simulink model "Version4"  (R2021a)
settings: Solver=VariableStepAuto  StartTime=0.0  StopTime=10.0  RelTol=1e-3
undefined symbols (not defined in the file): K, Lm, Lr, Rr, Rs
settings Model: Creator=shahk  LastModifiedBy=Aashish Kalra
settings OptimizationCC: UseDivisionForNetSlopeComputation=UseDivisionForReciprocalsOfIntegersOnly  DefaultUnderspecifiedDataType=single
settings DebuggingCC: SignalInfNanChecking=warning  UnconnectedInputMsg=none  UnconnectedOutputMsg=none  UnconnectedLineMsg=none  UniqueDataStoreMsg=error  AssertControl=DisableAll  StrictBusMsg=ErrorOnBusTreatedAsVector
settings SFSimCC: CompileTimeRecursionLimit=0  MATLABDynamicMemAlloc=off
settings RTWCC: DLArmComputeVersion=20.02.1
settings ConfigComp: CovEnable=on  CovScope=ReferencedModels  RecordCoverage=on  CovModelRefEnable=filtered

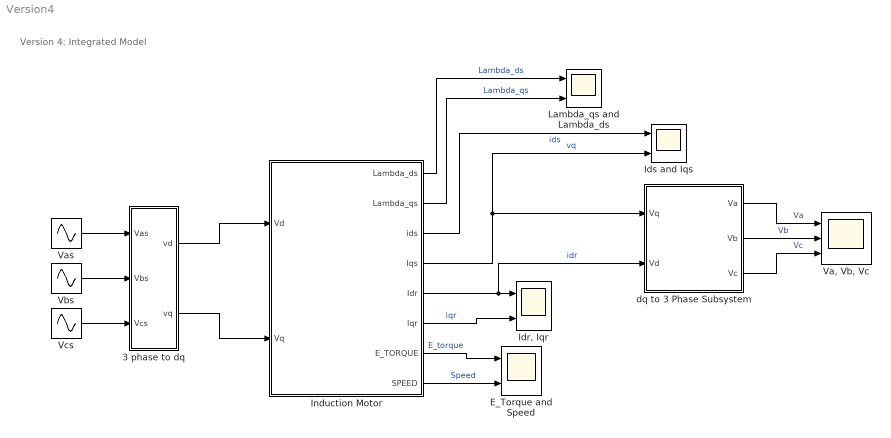
== system Version4 ==
  note: Version 4: Integrated Model
  3 phase to dq : Subsystem
  E_Torque and Speed : Scope  NumInputPorts=2
  "Idr, Iqr" : Scope  NumInputPorts=2
  Ids and Iqs : Scope  NumInputPorts=2
  Induction Motor : Subsystem
  Lambda_qs and Lambda_ds : Scope  NumInputPorts=2
  "Va, Vb, Vc" : Scope  NumInputPorts=3
  Vas : Sin  Amplitude=220*sqrt(2)  Frequency=2*pi*60  Phase=(pi/2)  SampleTime=0
  Vbs : Sin  Amplitude=220*sqrt(2)  Frequency=2*pi*60  Phase=((-2*pi)/3)+(pi/2)  SampleTime=0
  Vcs : Sin  Amplitude=220*sqrt(2)  Frequency=2*pi*60  Phase=((2*pi)/3)+(pi/2)  SampleTime=0
  dq to 3 Phase Subsystem : Subsystem
  wires:
  Induction Motor/6(Iqr) -> "Idr, Iqr"/2  "iqr"
  dq to 3 Phase Subsystem/1(Va) -> "Va, Vb, Vc"/1  "Va"
  dq to 3 Phase Subsystem/3(Vc) -> "Va, Vb, Vc"/3  "Vc"
  Induction Motor/4(Iqs) -> Ids and Iqs/2, dq to 3 Phase Subsystem/1(Vq)  "vq"
  Induction Motor/2(Lambda_qs) -> Lambda_qs and Lambda_ds/2  "Lambda_qs"
  dq to 3 Phase Subsystem/2(Vb) -> "Va, Vb, Vc"/2  "Vb"
  Induction Motor/3(ids) -> Ids and Iqs/1  "ids"
  Induction Motor/8(SPEED) -> E_Torque and Speed/2  "Speed"
  3 phase to dq/2(vq) -> Induction Motor/2(Vq)
  3 phase to dq/1(vd) -> Induction Motor/1(Vd)
  Induction Motor/7("E_TORQUE ") -> E_Torque and Speed/1  "E_torque"
  Induction Motor/5(Idr) -> dq to 3 Phase Subsystem/2(Vd), "Idr, Iqr"/1  "idr"
  Induction Motor/1(Lambda_ds) -> Lambda_qs and Lambda_ds/1  "Lambda_ds"
  Vas/1 -> 3 phase to dq/1(Vas)
  Vbs/1 -> 3 phase to dq/2(Vbs)
  Vcs/1 -> 3 phase to dq/3(Vcs)

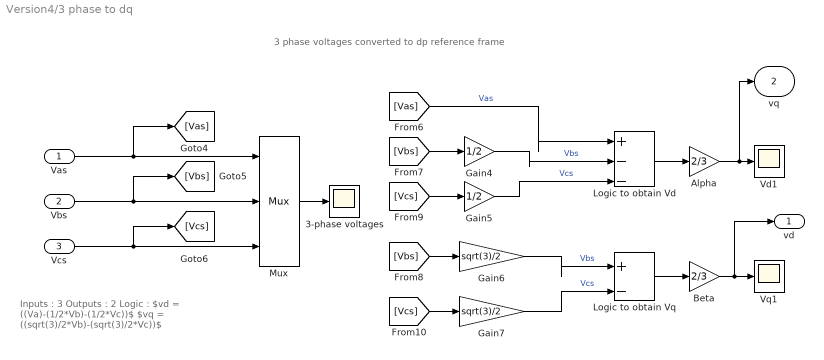
== system Version4/3 phase to dq ==
  note: Inputs : 3
      | Outputs : 2
      |
      | Logic :
      | $vd = ((Va)-(1/2*Vb)-(1/2*Vc))$
      | $vq = ((sqrt(3)/2*Vb)-(sqrt(3)/2*Vc))$
  note: 3 phase voltages converted to dp reference frame
  Vas : Inport
  Vbs : Inport  Port=2
  Vcs : Inport  Port=3
  3-phase voltages : Scope
  Alpha : Gain  Gain=2/3
  Beta : Gain  Gain=2/3
  Gain4 : Gain  Gain=1/2
  Gain5 : Gain  Gain=1/2
  Gain6 : Gain  Gain=sqrt(3)/2
  Gain7 : Gain  Gain=sqrt(3)/2
  Logic to obtain Vd : Sum  Inputs=|+--
  Logic to obtain Vq : Sum  Inputs=|+-
  Mux : Mux  Inputs=3
  Vd1 : Scope
  Vq1 : Scope
  vd : Outport
  vq : Outport  Port=2
  wires:
  Gain4/1 -> Logic to obtain Vd/2  "Vbs"
  Gain7/1 -> Logic to obtain Vq/2  "Vcs"
  [Vcs] -> Gain5/1
  Vcs/1 -> [Vcs], Mux/3
  Vbs/1 -> [Vbs], Mux/2
  [Vas] -> Logic to obtain Vd/1  "Vas"
  Vas/1 -> [Vas], Mux/1
  Logic to obtain Vq/1 -> Beta/1
  [Vcs] -> Gain7/1
  Gain6/1 -> Logic to obtain Vq/1  "Vbs"
  [Vbs] -> Gain6/1
  [Vbs] -> Gain4/1
  Logic to obtain Vd/1 -> Alpha/1
  Gain5/1 -> Logic to obtain Vd/3  "Vcs"
  Beta/1 -> vd/1, Vq1/1
  Mux/1 -> 3-phase voltages/1
  Alpha/1 -> vq/1, Vd1/1

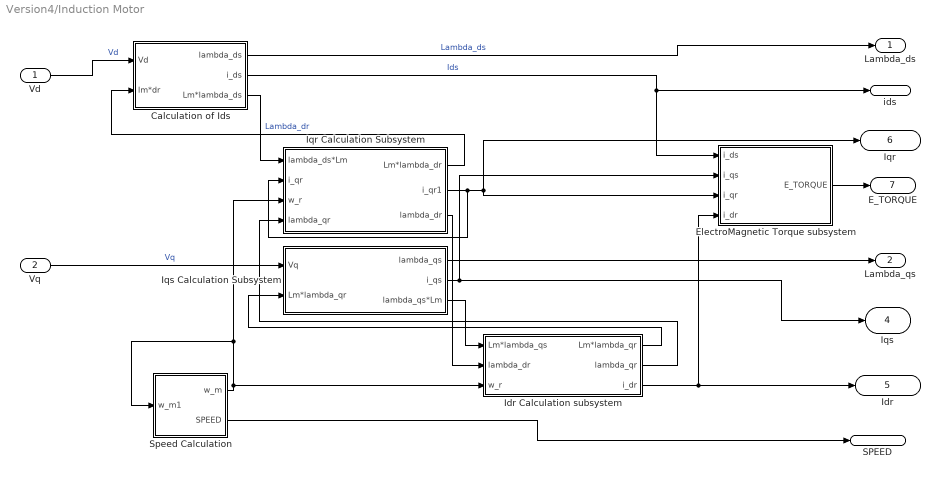
== system Version4/Induction Motor ==
  Vd : Inport
  Vq : Inport  Port=2
  Calculation of Ids : Subsystem
  ElectroMagnetic Torque subsystem : Subsystem
  Idr Calculation subsystem : Subsystem
  Iqr Calculation Subsystem : Subsystem
  Iqs Calculation Subsystem : Subsystem
  Speed Calculation : Subsystem
  Lambda_ds : Outport  VectorParamsAs1DForOutWhenUnconnected=off
  Lambda_qs : Outport  Port=2  VectorParamsAs1DForOutWhenUnconnected=off
  ids : Outport  Port=3  VectorParamsAs1DForOutWhenUnconnected=off
  Iqs : Outport  Port=4  VectorParamsAs1DForOutWhenUnconnected=off
  Idr : Outport  Port=5  VectorParamsAs1DForOutWhenUnconnected=off
  Iqr : Outport  Port=6  VectorParamsAs1DForOutWhenUnconnected=off
  "E_TORQUE " : Outport  Port=7  VectorParamsAs1DForOutWhenUnconnected=off
  SPEED : Outport  Port=8  VectorParamsAs1DForOutWhenUnconnected=off
  wires:
  Idr Calculation subsystem/2(lambda_qr) -> Iqr Calculation Subsystem/4(lambda_qr)
  ElectroMagnetic Torque subsystem/1("E_TORQUE ") -> "E_TORQUE "/1
  Speed Calculation/2(SPEED) -> SPEED/1
  Idr Calculation subsystem/1(Lm*lambda_qr) -> Iqs Calculation Subsystem/2(Lm*lambda_qr)
  Iqr Calculation Subsystem/1(Lm*lambda_dr) -> Calculation of Ids/2(lm*dr)  "Lambda_dr"
  Iqs Calculation Subsystem/3(lambda_qs*Lm) -> Idr Calculation subsystem/1(Lm*lambda_qs)
  Iqr Calculation Subsystem/3(lambda_dr) -> Idr Calculation subsystem/2(lambda_dr)
  Iqs Calculation Subsystem/1(lambda_qs) -> Lambda_qs/1
  Vq/1 -> Iqs Calculation Subsystem/1(Vq)  "Vq"
  Vd/1 -> Calculation of Ids/1(Vd)  "Vd"
  Calculation of Ids/1(lambda_ds) -> Lambda_ds/1  "Lambda_ds"
  Calculation of Ids/3(Lm*lambda_ds) -> Iqr Calculation Subsystem/1(lambda_ds*Lm)
  Speed Calculation/1(w_m) -> Speed Calculation/1(w_m1), Iqr Calculation Subsystem/3(w_r), Idr Calculation subsystem/3(w_r)
  Idr Calculation subsystem/3(i_dr) -> ElectroMagnetic Torque subsystem/4(i_dr), Idr/1
  Iqr Calculation Subsystem/2(i_qr1) -> ElectroMagnetic Torque subsystem/3(i_qr), Iqr/1, Iqr Calculation Subsystem/2(i_qr)
  Iqs Calculation Subsystem/2(i_qs) -> Iqs/1, ElectroMagnetic Torque subsystem/2(i_qs)
  Calculation of Ids/2(i_ds) -> ElectroMagnetic Torque subsystem/1(i_ds), ids/1  "Ids"

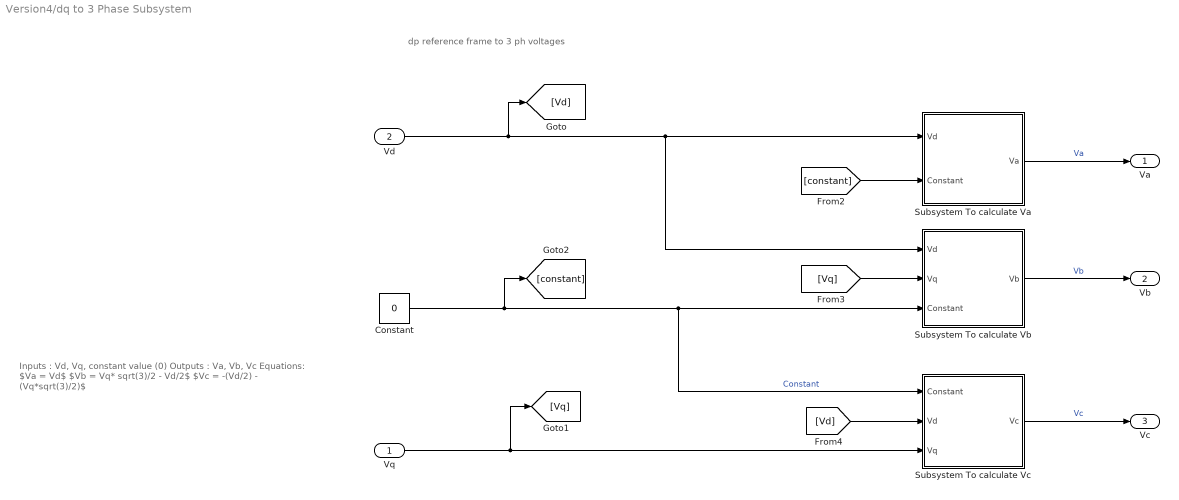
== system Version4/dq to 3 Phase Subsystem ==
  note: Inputs : Vd, Vq, constant value (0)
      | Outputs : Va, Vb, Vc
      |
      | Equations:
      |
      | $Va = Vd$
      | $Vb = Vq* sqrt(3)/2 - Vd/2$
      | $Vc = -(Vd/2) - (Vq*sqrt(3)/2)$
  note: dp reference frame to 3 ph voltages
  Vq : Inport
  Vd : Inport  Port=2
  Constant : Constant  Value=0
  Subsystem To calculate Va : Subsystem
  Subsystem To calculate Vb : Subsystem
  Subsystem To calculate Vc : Subsystem
  Va : Outport  VectorParamsAs1DForOutWhenUnconnected=off
  Vb : Outport  Port=2  VectorParamsAs1DForOutWhenUnconnected=off
  Vc : Outport  Port=3  VectorParamsAs1DForOutWhenUnconnected=off
  wires:
  [constant] -> Subsystem To calculate Va/2(Constant)
  Subsystem To calculate Va/1(Va) -> Va/1  "Va"
  Subsystem To calculate Vc/1(Vc) -> Vc/1  "Vc"
  [Vq] -> Subsystem To calculate Vb/2(Vq)
  Constant/1 -> [constant], Subsystem To calculate Vc/1(Constant), Subsystem To calculate Vb/3(Constant)  "Constant"
  Vq/1 -> [Vq], Subsystem To calculate Vc/3(Vq)
  Vd/1 -> [Vd], Subsystem To calculate Vb/1(Vd), Subsystem To calculate Va/1(Vd)
  [Vd] -> Subsystem To calculate Vc/2(Vd)
  Subsystem To calculate Vb/1(Vb) -> Vb/1  "Vb"

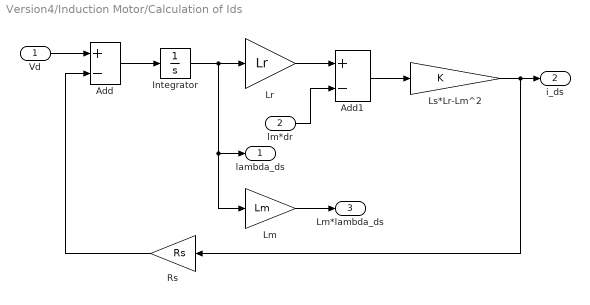
== system Version4/Induction Motor/Calculation of Ids ==
  Vd : Inport
  lm*dr : Inport  Port=2
  Add : Sum  Inputs=+-
  Add1 : Sum  Inputs=+-
  Integrator : Integrator
  Lm : Gain  Gain=Lm
  Lr : Gain  Gain=Lr
  Ls*Lr-Lm^2 : Gain  Gain=K
  Rs : Gain  Gain=Rs
  lambda_ds : Outport  VectorParamsAs1DForOutWhenUnconnected=off
  i_ds : Outport  Port=2
  Lm*lambda_ds : Outport  Port=3
  wires:
  Ls*Lr-Lm^2/1 -> Rs/1, i_ds/1
  lm*dr/1 -> Add1/2
  Lr/1 -> Add1/1
  Add1/1 -> Ls*Lr-Lm^2/1
  Lm/1 -> Lm*lambda_ds/1
  Add/1 -> Integrator/1
  Vd/1 -> Add/1
  Rs/1 -> Add/2
  Integrator/1 -> lambda_ds/1, Lm/1, Lr/1

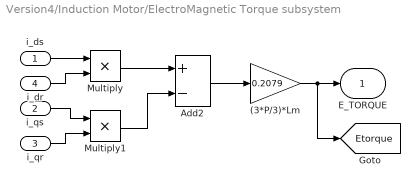
== system Version4/Induction Motor/ElectroMagnetic Torque subsystem ==
  i_ds : Inport
  i_qs : Inport  Port=2
  i_qr : Inport  Port=3
  i_dr : Inport  Port=4
  (3*P/3)*Lm : Gain  Gain=0.2079
  Add2 : Sum  Inputs=+-
  Multiply : Product
  Multiply1 : Product
  "E_TORQUE " : Outport  VectorParamsAs1DForOutWhenUnconnected=off
  tag scope: Etorque=global
  wires:
  (3*P/3)*Lm/1 -> [Etorque], "E_TORQUE "/1
  i_qs/1 -> Multiply1/1
  i_dr/1 -> Multiply/2
  Multiply/1 -> Add2/1
  Add2/1 -> (3*P/3)*Lm/1
  i_qr/1 -> Multiply1/2
  i_ds/1 -> Multiply/1
  Multiply1/1 -> Add2/2

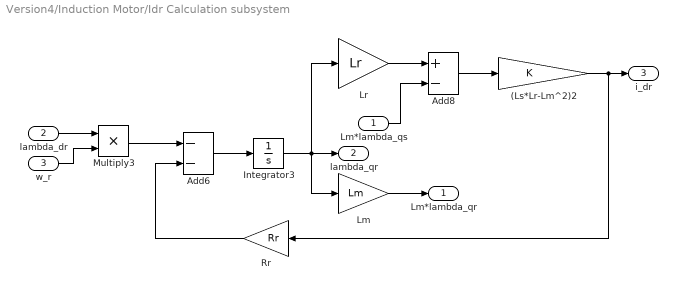
== system Version4/Induction Motor/Idr Calculation subsystem ==
  Lm*lambda_qs : Inport
  lambda_dr : Inport  Port=2
  w_r : Inport  Port=3
  (Ls*Lr-Lm^2)2 : Gain  Gain=K
  Add6 : Sum  Inputs=--
  Add8 : Sum  Inputs=+-
  Integrator3 : Integrator
  Lm : Gain  Gain=Lm
  Lr : Gain  Gain=Lr
  Multiply3 : Product
  Rr : Gain  Gain=Rr
  Lm*lambda_qr : Outport
  lambda_qr : Outport  Port=2
  i_dr : Outport  Port=3
  wires:
  Rr/1 -> Add6/2
  Add6/1 -> Integrator3/1
  lambda_dr/1 -> Multiply3/1
  Lm*lambda_qs/1 -> Add8/2
  Lr/1 -> Add8/1
  Add8/1 -> (Ls*Lr-Lm^2)2/1
  Lm/1 -> Lm*lambda_qr/1
  w_r/1 -> Multiply3/2
  Multiply3/1 -> Add6/1
  Integrator3/1 -> lambda_qr/1, Lm/1, Lr/1
  (Ls*Lr-Lm^2)2/1 -> i_dr/1, Rr/1

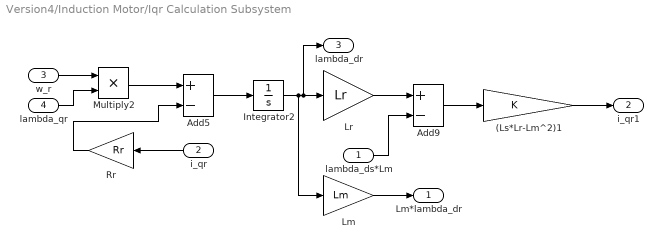
== system Version4/Induction Motor/Iqr Calculation Subsystem ==
  lambda_ds*Lm : Inport
  i_qr : Inport  Port=2
  w_r : Inport  Port=3
  lambda_qr : Inport  Port=4
  (Ls*Lr-Lm^2)1 : Gain  Gain=K
  Add5 : Sum  Inputs=+-
  Add9 : Sum  Inputs=+-
  Integrator2 : Integrator
  Lm : Gain  Gain=Lm
  Lr : Gain  Gain=Lr
  Multiply2 : Product
  Rr : Gain  Gain=Rr
  Lm*lambda_dr : Outport
  i_qr1 : Outport  Port=2
  lambda_dr : Outport  Port=3
  wires:
  Rr/1 -> Add5/2
  Multiply2/1 -> Add5/1
  w_r/1 -> Multiply2/1
  lambda_ds*Lm/1 -> Add9/2
  Lr/1 -> Add9/1
  i_qr/1 -> Rr/1
  (Ls*Lr-Lm^2)1/1 -> i_qr1/1
  lambda_qr/1 -> Multiply2/2
  Lm/1 -> Lm*lambda_dr/1
  Add9/1 -> (Ls*Lr-Lm^2)1/1
  Add5/1 -> Integrator2/1
  Integrator2/1 -> lambda_dr/1, Lr/1, Lm/1

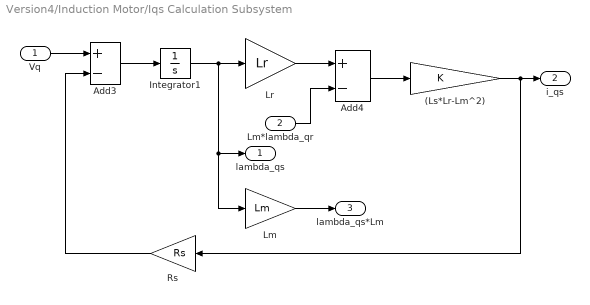
== system Version4/Induction Motor/Iqs Calculation Subsystem ==
  Vq : Inport
  Lm*lambda_qr : Inport  Port=2
  (Ls*Lr-Lm^2) : Gain  Gain=K
  Add3 : Sum  Inputs=+-
  Add4 : Sum  Inputs=+-
  Integrator1 : Integrator
  Lm : Gain  Gain=Lm
  Lr : Gain  Gain=Lr
  Rs : Gain  Gain=Rs
  lambda_qs : Outport  VectorParamsAs1DForOutWhenUnconnected=off
  i_qs : Outport  Port=2
  lambda_qs*Lm : Outport  Port=3
  wires:
  (Ls*Lr-Lm^2)/1 -> Rs/1, i_qs/1
  Lr/1 -> Add4/1
  Add4/1 -> (Ls*Lr-Lm^2)/1
  Lm*lambda_qr/1 -> Add4/2
  Rs/1 -> Add3/2
  Lm/1 -> lambda_qs*Lm/1
  Vq/1 -> Add3/1
  Add3/1 -> Integrator1/1
  Integrator1/1 -> lambda_qs/1, Lm/1, Lr/1

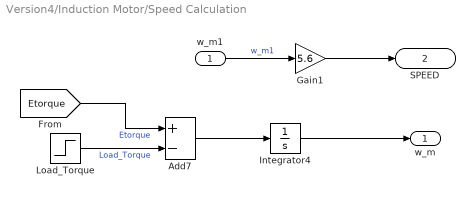
== system Version4/Induction Motor/Speed Calculation ==
  w_m1 : Inport
  Add7 : Sum  Inputs=+-
  Gain1 : Gain  Gain=5.6
  Integrator4 : Integrator
  Load_Torque : Step  Time=5  After=20  SampleTime=0
  w_m : Outport
  SPEED : Outport  Port=2  VectorParamsAs1DForOutWhenUnconnected=off
  wires:
  w_m1/1 -> Gain1/1  "w_m1"
  Integrator4/1 -> w_m/1
  [Etorque] -> Add7/1  "Etorque"
  Gain1/1 -> SPEED/1
  Add7/1 -> Integrator4/1
  Load_Torque/1 -> Add7/2  "Load_Torque"

== system Version4/dq to 3 Phase Subsystem/Subsystem To calculate Va ==
  Vd : Inport
  Constant : Inport  Port=2
  Gain6 : Gain
  Gain9 : Gain
  Logic for Va : Sum  Inputs=|++
  Va : Outport
  wires:
  Vd/1 -> Gain6/1  "Vd"
  Constant/1 -> Gain9/1  "Constant"
  Gain6/1 -> Logic for Va/1
  Gain9/1 -> Logic for Va/2
  Logic for Va/1 -> Va/1

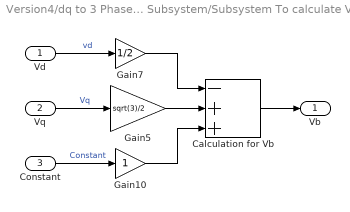
== system Version4/dq to 3 Phase Subsystem/Subsystem To calculate Vb ==
  Vd : Inport
  Vq : Inport  Port=2
  Constant : Inport  Port=3
  Calculation for Vb : Sum  Inputs=-++
  Gain10 : Gain
  Gain5 : Gain  Gain=sqrt(3)/2
  Gain7 : Gain  Gain=1/2
  Vb : Outport
  wires:
  Vq/1 -> Gain5/1  "Vq"
  Vd/1 -> Gain7/1  "vd"
  Constant/1 -> Gain10/1  "Constant"
  Gain7/1 -> Calculation for Vb/1
  Calculation for Vb/1 -> Vb/1
  Gain10/1 -> Calculation for Vb/3
  Gain5/1 -> Calculation for Vb/2

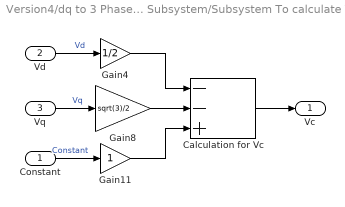
== system Version4/dq to 3 Phase Subsystem/Subsystem To calculate Vc ==
  Constant : Inport
  Vd : Inport  Port=2
  Vq : Inport  Port=3
  Calculation for Vc : Sum  Inputs=--+
  Gain11 : Gain
  Gain4 : Gain  Gain=1/2
  Gain8 : Gain  Gain=sqrt(3)/2
  Vc : Outport
  wires:
  Constant/1 -> Gain11/1  "Constant"
  Gain11/1 -> Calculation for Vc/3
  Calculation for Vc/1 -> Vc/1
  Vd/1 -> Gain4/1  "Vd"
  Gain4/1 -> Calculation for Vc/1
  Gain8/1 -> Calculation for Vc/2
  Vq/1 -> Gain8/1  "Vq"
